simulink model "TwoTanks_PID_R2018a"  (R2018a)
settings: Solver=ode4  StartTime=0.0  StopTime=tfinal  FixedStep=dt  RelTol=1e-3  EnableMultiTasking=on
values from neighbouring files (symbols this model uses):
  a1 = 0.0190125110732    [GWO_workspace_PID.mat]    (also in GWO_workspace_PID_v1.1.mat; GWO_workspace_PID_v1.2.mat; GWO_workspace_PID_v1.3.mat; GWO_workspace_PID_v1.4.mat)
  a2 = 0.594107643424    [GWO_workspace_PID.mat]    (also in GWO_workspace_PID_v1.1.mat; GWO_workspace_PID_v1.2.mat; GWO_workspace_PID_v1.3.mat; GWO_workspace_PID_v1.4.mat)
  a3 = 0.0893725569407    [GWO_workspace_PID.mat]    (also in GWO_workspace_PID_v1.1.mat; GWO_workspace_PID_v1.2.mat; GWO_workspace_PID_v1.3.mat; GWO_workspace_PID_v1.4.mat)
  a4 = 0.0670294177055    [GWO_workspace_PID.mat]    (also in GWO_workspace_PID_v1.1.mat; GWO_workspace_PID_v1.2.mat; GWO_workspace_PID_v1.3.mat; GWO_workspace_PID_v1.4.mat)
  h10 = 0.1    [GWO_workspace_PID.mat]    (also in GWO_workspace_PID_v1.1.mat; GWO_workspace_PID_v1.2.mat; GWO_workspace_PID_v1.3.mat; GWO_workspace_PID_v1.4.mat)
  H1max = 1    [GWO_workspace_PID.mat]    (also in GWO_workspace_PID_v1.1.mat; GWO_workspace_PID_v1.2.mat; GWO_workspace_PID_v1.3.mat; GWO_workspace_PID_v1.4.mat)
  h20 = 0.1    [GWO_workspace_PID.mat]    (also in GWO_workspace_PID_v1.1.mat; GWO_workspace_PID_v1.2.mat; GWO_workspace_PID_v1.3.mat; GWO_workspace_PID_v1.4.mat)
  H2max = 1    [GWO_workspace_PID.mat]    (also in GWO_workspace_PID_v1.1.mat; GWO_workspace_PID_v1.2.mat; GWO_workspace_PID_v1.3.mat; GWO_workspace_PID_v1.4.mat)
  kD = 8.55422602032    [GWO_workspace_PID.mat]    (also in GWO_workspace_PID_v1.1.mat = 1.07531549365; GWO_workspace_PID_v1.2.mat = 1.23039074493; GWO_workspace_PID_v1.3.mat = 1.23039074493; GWO_workspace_PID_v1.4.mat = 1.09650188431)
  kI = 10.3156904646    [GWO_workspace_PID.mat]    (also in GWO_workspace_PID_v1.1.mat = 12.6462667539; GWO_workspace_PID_v1.2.mat = 10.3199209754; GWO_workspace_PID_v1.3.mat = 10.3199209754; GWO_workspace_PID_v1.4.mat = 19.9449136043)
  kP = 70.3203061082    [GWO_workspace_PID.mat]    (also in GWO_workspace_PID_v1.1.mat = 58.4171274691; GWO_workspace_PID_v1.2.mat = 59.6465103347; GWO_workspace_PID_v1.3.mat = 59.6465103347; GWO_workspace_PID_v1.4.mat = 148.223544056)
  satF_inf = 10    [GWO_workspace_PID.mat]    (also in GWO_workspace_PID_v1.1.mat; GWO_workspace_PID_v1.2.mat; GWO_workspace_PID_v1.3.mat; GWO_workspace_PID_v1.4.mat)
  satF_sup = 90    [GWO_workspace_PID.mat]    (also in GWO_workspace_PID_v1.1.mat; GWO_workspace_PID_v1.2.mat; GWO_workspace_PID_v1.3.mat; GWO_workspace_PID_v1.4.mat)
libraries: simulink x1
settings Model: Creator=joniram  LastModifiedBy=generic-user
settings DataIOCC: ExternalInput=[limV1F_sup, limV1F_inf, limV2F_sup, limV2F_inf]  LimitDataPoints=on  SaveFormat=Array  SignalLoggingSaveFormat=ModelDataLogs
settings OptimizationCC: ExpressionDepthLimit=2147483647  LifeSpan=inf
settings DebuggingCC: UnderspecifiedInitializationDetection=Classic  MergeDetectMultiDrivingBlocksExec=none  SolverPrmCheckMsg=warning  FcnCallInpInsideContextMsg=warning  StateNameClashWarn=warning  SFUnexpectedBacktrackingDiag=warning  SFNoUnconditionalDefaultTransitionDiag=warning  SFExecutionAtInitializationDiag=none
settings HardwareCC: ProdBitPerPointer=32  ProdBitPerSizeT=32  ProdBitPerPtrDiffT=32  ProdLargestAtomicFloat=None  ProdIntDivRoundTo=Undefined  ProdEndianess=Unspecified  ProdWordSize=32  ProdHWDeviceType=32-bit Generic
settings ModelReferenceCC: PropagateSignalLabelsOutOfModel=off
settings CodeAppCC: StateflowObjectComments=on
settings GRTTargetCC: TargetLangStandard=C89/C90 (ANSI)  GeneratePreprocessorConditionals=Disable all  CombineOutputUpdateFcns=off  GRTInterface=on
settings ConfigComp: CovMetricSettings=dw  CovHtmlReporting=on  CovSaveCumulativeToWorkspaceVar=on  CovSaveSingleToWorkspaceVar=on  CovExternalEMLEnable=off

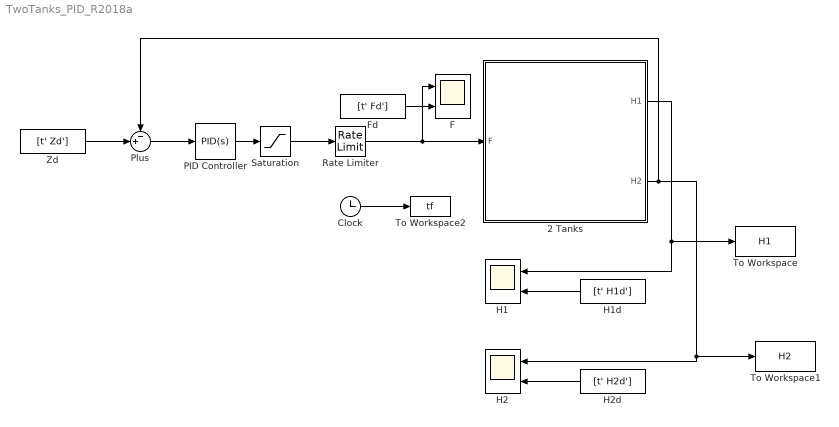
== system TwoTanks_PID_R2018a ==
  2 Tanks : Subsystem
  Clock : Clock
  F : Scope  NumInputPorts=2
  Fd : FromWorkspace  VariableName=[t' Fd']  SampleTime=0  OutputAfterFinalValue=Holding final value
  H1 : Scope  NumInputPorts=2
  H1d : FromWorkspace  VariableName=[t' H1d']  SampleTime=0  OutputAfterFinalValue=Holding final value
  H2 : Scope  NumInputPorts=2
  H2d : FromWorkspace  VariableName=[t' H2d']  SampleTime=0  OutputAfterFinalValue=Holding final value
  PID Controller : simulink/Continuous/PID Controller  Controller=PID  TimeDomain=Continuous-time  SampleTime=-1  IntegratorMethod=Forward Euler  FilterMethod=Forward Euler  Form=Parallel  UseFilter=on  ControllerParametersSource=internal  P=kP  I=kI  D=kD  N=100  InitialConditionSource=internal  InitialConditionForIntegrator=0  InitialConditionForFilter=0  ExternalReset=none  LimitOutput=off  UpperSaturationLimit=inf  LowerSaturationLimit=-inf  LinearizeAsGain=on  AntiWindupMode=none  Kb=1  TrackingMode=off  Kt=1  PParamMin=[]  PParamMax=[]  IParamMin=[]  IParamMax=[]  DParamMin=[]  DParamMax=[]  NParamMin=[]  NParamMax=[]  KbParamMin=[]  KbParamMax=[]  KtParamMin=[]  KtParamMax=[]  POutMin=[]  POutMax=[]  IOutMin=[]  IOutMax=[]  DOutMin=[]  DOutMax=[]  NOutMin=[]  NOutMax=[]  KbOutMin=[]  KbOutMax=[]  KtOutMin=[]  KtOutMax=[]  IntegratorOutMin=[]  IntegratorOutMax=[]  FilterOutMin=[]  FilterOutMax=[]  SumOutMin=[]  SumOutMax=[]  SumI1OutMin=[]  SumI1OutMax=[]  SumI2OutMin=[]  SumI2OutMax=[]  SumI3OutMin=[]  SumI3OutMax=[]  SumDOutMin=[]  SumDOutMax=[]  SaturationOutMin=[]  SaturationOutMax=[]  IntegratorContinuousStateAttributes=''  IntegratorStateMustResolveToSignalObject=off  IntegratorRTWStateStorageClass=Auto  FilterContinuousStateAttributes=''  FilterStateMustResolveToSignalObject=off  FilterRTWStateStorageClass=Auto  DifferentiatorICPrevScaledInput=0  DifferentiatorOutMin=[]  DifferentiatorOutMax=[]  FilterDiffOutCoefMin=[]  FilterDiffOutCoefMax=[]  SumDenOutMin=[]  SumDenOutMax=[]  SumNumOutMin=[]  SumNumOutMax=[]  ReciprocalOutMin=[]  ReciprocalOutMax=[]  DivideOutMin=[]  DivideOutMax=[]  TunerSelectOption=Transfer Function Based (PID Tuner App)
  Plus : Sum  Inputs=-+|
  Rate Limiter : RateLimiter  RisingSlewLimit=200  FallingSlewLimit=-200  SampleTimeMode=inherited
  Saturation : Saturate  UpperLimit=satF_sup  LowerLimit=satF_inf
  To Workspace : ToWorkspace  VariableName=H1  SampleTime=-1
  To Workspace1 : ToWorkspace  VariableName=H2  SampleTime=-1
  To Workspace2 : ToWorkspace  VariableName=tf  SampleTime=-1
  Zd : FromWorkspace  VariableName=[t' Zd']  SampleTime=0  OutputAfterFinalValue=Holding final value
  wires:
  2 Tanks/2(H2) -> To Workspace1/1, H2/1, Plus/1
  2 Tanks/1(H1) -> To Workspace/1, H1/1
  PID Controller/1 -> Saturation/1
  H2d/1 -> H2/2
  Clock/1 -> To Workspace2/1
  H1d/1 -> H1/2
  Fd/1 -> F/2
  Plus/1 -> PID Controller/1
  Zd/1 -> Plus/2
  Saturation/1 -> Rate Limiter/1
  Rate Limiter/1 -> F/1, 2 Tanks/1(F)

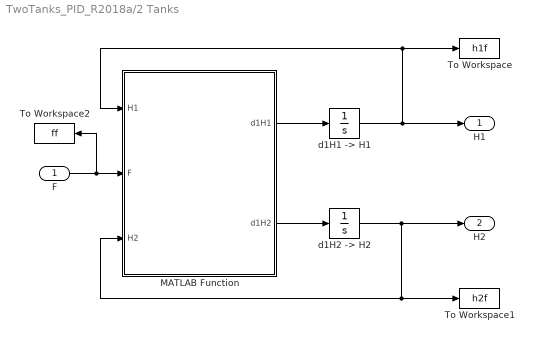
== system TwoTanks_PID_R2018a/2 Tanks ==
  F : Inport
  MATLAB Function : MATLAB Function  TreatAsAtomicUnit=on
  To Workspace : ToWorkspace  VariableName=h1f  SampleTime=-1
  To Workspace1 : ToWorkspace  VariableName=h2f  SampleTime=-1
  To Workspace2 : ToWorkspace  VariableName=ff  SampleTime=-1
  "d1H1 -> H1" : Integrator  InitialCondition=h10  LimitOutput=on  UpperSaturationLimit=H1max  LowerSaturationLimit=0
  "d1H2 -> H2" : Integrator  InitialCondition=h20  LimitOutput=on  UpperSaturationLimit=H2max  LowerSaturationLimit=0
  H1 : Outport
  H2 : Outport  Port=2
  wires:
  MATLAB Function/1(d1H1) -> "d1H1 -> H1"/1
  "d1H1 -> H1"/1 -> H1/1, To Workspace/1, MATLAB Function/1(H1)
  MATLAB Function/2(d1H2) -> "d1H2 -> H2"/1
  F/1 -> To Workspace2/1, MATLAB Function/2(F)
  "d1H2 -> H2"/1 -> H2/1, To Workspace1/1, MATLAB Function/3(H2)

== matlab function TwoTanks_PID_R2018a/2 Tanks/MATLAB Function ==
  data: H1 input; F input; d1H1 output; H2 input; d1H2 output; a1 parameter; a2 parameter; a3 parameter; a4 parameter
function [d1H1, d1H2] = TwoTanks(H1, F, H2, a1, a2, a3, a4)
  
  % Sistema Dinâmico
    d1H1 = a1*F - a2*sqrt(H1);
    
    d1H2 = a3*(sqrt(H1)/(H2^2)) - a4*(1/(H2^1.5));
